simulink model "complete_model"  (R2020b)
settings: Solver=VariableStepAuto  StartTime=0.0  StopTime=10.0  RelTol=1e-3
undefined symbols (not defined in the file or in its folder): D_b_1, D_b_2, D_k_1, D_k_2, D_t_1, D_t_2, E_1, E_2, g, Gs_1, Gs_2, Ix_1, Ix_2, Iy_1, Iy_2, Iz_1, Iz_2, l_1, l_2, m_1, m_2, q_0, q_dot_0
libraries: dspmtrx3 x2, pid_lib x1, dspinverses x1
(part 2 of 2)

== matlab function complete_model/CONTROLLER/Subsystem2/MATLAB Function2 ==
  data: g input; B_matrix output; Ix_1 input; Ix_2 input; Iy_1 input; Iy_2 input; Iz_1 input; Iz_2 input; b_1 input; b_2 input; b_dot_1 input; b_dot_2 input; k_1 input; k_2 input; k_dot_1 input; k_dot_2 input; l_1 input; l_2 input; m_1 input; m_2 input; t_1 input; t_2 input; t_dot_1 input; t_dot_2 input; E_1 input; E_2 input; Gs_1 input; Gs_2 input; G_matrix output; C_matrix output
function [B_matrix,G_matrix,C_matrix] = compute_matrixs(g,Ix_1,Ix_2,Iy_1,Iy_2,Iz_1,Iz_2,b_1,b_2,b_dot_1,b_dot_2,k_1,k_2,k_dot_1,k_dot_2,l_1,l_2,m_1,m_2,t_1,t_2,t_dot_1,t_dot_2,E_1,E_2,Gs_1,Gs_2)

C_11 = C11(Ix_1,Iy_1,Iz_1,b_1,b_2,b_dot_1,b_dot_2,k_1,k_2,k_dot_1,k_dot_2,l_1,l_2,m_1,t_1,t_2,t_dot_1,t_dot_2);
C_12 = C12(Ix_1,Iy_1,Iz_1,b_1,b_2,b_dot_1,b_dot_2,k_1,k_2,k_dot_1,k_dot_2,l_1,l_2,m_1,t_1,t_2,t_dot_1,t_dot_2);
C_13 = C13(Ix_1,Iy_1,Iz_1,b_1,b_2,b_dot_1,b_dot_2,k_1,k_2,k_dot_1,k_dot_2,l_1,l_2,m_1,t_1,t_2,t_dot_1,t_dot_2);
C_14 = C14(Ix_1,Ix_2,Iy_1,Iy_2,Iz_1,Iz_2,b_1,b_2,b_dot_1,b_dot_2,k_1,k_2,k_dot_1,k_dot_2,l_1,l_2,m_1,m_2,t_1,t_2,t_dot_1,t_dot_2);
C_15 = C15(Ix_1,Ix_2,Iy_1,Iy_2,Iz_1,Iz_2,b_1,b_2,b_dot_1,b_dot_2,k_1,k_2,k_dot_1,k_dot_2,l_1,l_2,m_1,m_2,t_1,t_2,t_dot_1,t_dot_2);
C_16 = C16(Ix_1,Ix_2,Iy_1,Iy_2,Iz_1,Iz_2,b_1,b_2,b_dot_1,b_dot_2,k_1,k_2,k_dot_1,k_dot_2,l_1,l_2,m_1,m_2,t_1,t_2,t_dot_1,t_dot_2);

C_21 = C21(Ix_1,Iy_1,Iz_1,b_1,b_2,b_dot_1,b_dot_2,k_1,k_2,k_dot_1,k_dot_2,l_1,l_2,m_1,t_1,t_2,t_dot_1,t_dot_2);
C_22 = C22(Ix_1,Iy_1,Iz_1,b_1,b_2,b_dot_1,b_dot_2,k_1,k_2,k_dot_1,k_dot_2,l_1,l_2,m_1,t_1,t_2,t_dot_1,t_dot_2);
C_23 = C23(Ix_1,Iy_1,Iz_1,b_1,b_2,b_dot_1,b_dot_2,k_1,k_2,k_dot_1,k_dot_2,l_1,l_2,m_1,t_1,t_2,t_dot_1,t_dot_2);
C_24 = C24(Ix_1,Ix_2,Iy_1,Iy_2,Iz_1,Iz_2,b_1,b_2,b_dot_1,b_dot_2,k_1,k_2,k_dot_1,k_dot_2,l_1,l_2,m_1,m_2,t_1,t_2,t_dot_1,t_dot_2);
C_25 = C25(Ix_1,Ix_2,Iy_1,Iy_2,Iz_1,Iz_2,b_1,b_2,b_dot_1,b_dot_2,k_1,k_2,k_dot_1,k_dot_2,l_1,l_2,m_1,m_2,t_1,t_2,t_dot_1,t_dot_2);
C_26 = C26(Ix_1,Ix_2,Iy_1,Iy_2,Iz_1,Iz_2,b_1,b_2,b_dot_1,b_dot_2,k_1,k_2,k_dot_1,k_dot_2,l_1,l_2,m_1,m_2,t_1,t_2,t_dot_1,t_dot_2);

C_31 = C31(Ix_1,Iy_1,Iz_1,b_1,b_2,b_dot_1,b_dot_2,k_1,k_2,k_dot_1,k_dot_2,l_1,l_2,m_1,t_1,t_2,t_dot_1,t_dot_2);
C_32 = C32(Ix_1,Iy_1,Iz_1,b_1,b_2,b_dot_1,b_dot_2,k_1,k_2,k_dot_1,k_dot_2,l_1,l_2,m_1,t_1,t_2,t_dot_1,t_dot_2);
C_33 = C33(Ix_1,Iy_1,Iz_1,b_1,b_2,b_dot_1,b_dot_2,k_1,k_2,k_dot_1,k_dot_2,l_1,l_2,m_1,t_1,t_2,t_dot_1,t_dot_2);
C_34 = C34(Ix_1,Ix_2,Iy_1,Iy_2,Iz_1,Iz_2,b_1,b_2,b_dot_1,b_dot_2,k_1,k_2,k_dot_1,k_dot_2,l_1,l_2,m_1,m_2,t_1,t_2,t_dot_1,t_dot_2);
C_35 = C35(Ix_1,Ix_2,Iy_1,Iy_2,Iz_1,Iz_2,b_1,b_2,b_dot_1,b_dot_2,k_1,k_2,k_dot_1,k_dot_2,l_1,l_2,m_1,m_2,t_1,t_2,t_dot_1,t_dot_2);
C_36 = C36(Ix_1,Ix_2,Iy_1,Iy_2,Iz_1,Iz_2,b_1,b_2,b_dot_1,b_dot_2,k_1,k_2,k_dot_1,k_dot_2,l_1,l_2,m_1,m_2,t_1,t_2,t_dot_1,t_dot_2);

C_41 = C41(Ix_1,Ix_2,Iy_1,Iy_2,Iz_1,Iz_2,b_1,b_2,b_dot_1,b_dot_2,k_1,k_2,k_dot_1,k_dot_2,l_1,l_2,m_1,m_2,t_1,t_2,t_dot_1,t_dot_2);
C_42 = C42(Ix_1,Ix_2,Iy_1,Iy_2,Iz_1,Iz_2,b_1,b_2,b_dot_1,b_dot_2,k_1,k_2,k_dot_1,k_dot_2,l_1,l_2,m_1,m_2,t_1,t_2,t_dot_1,t_dot_2);
C_43 = C43(Ix_1,Ix_2,Iy_1,Iy_2,Iz_1,Iz_2,b_1,b_2,b_dot_1,b_dot_2,k_1,k_2,k_dot_1,k_dot_2,l_1,l_2,m_1,m_2,t_1,t_2,t_dot_1,t_dot_2);
C_44 = C44(Ix_2,Iy_2,Iz_2,b_1,b_2,b_dot_1,b_dot_2,k_1,k_2,k_dot_1,k_dot_2,l_1,l_2,m_2,t_1,t_2,t_dot_1,t_dot_2);
C_45 = C45(Ix_2,Iy_2,Iz_2,b_1,b_2,b_dot_1,b_dot_2,k_1,k_2,k_dot_1,k_dot_2,l_1,l_2,m_2,t_1,t_2,t_dot_1,t_dot_2);
C_46 = C46(Ix_2,Iy_2,Iz_2,b_1,b_2,b_dot_1,b_dot_2,k_1,k_2,k_dot_1,k_dot_2,l_1,l_2,m_2,t_1,t_2,t_dot_1,t_dot_2);

C_51 = C51(Ix_1,Ix_2,Iy_1,Iy_2,Iz_1,Iz_2,b_1,b_2,b_dot_1,b_dot_2,k_1,k_2,k_dot_1,k_dot_2,l_1,l_2,m_1,m_2,t_1,t_2,t_dot_1,t_dot_2);
C_52 = C52(Ix_1,Ix_2,Iy_1,Iy_2,Iz_1,Iz_2,b_1,b_2,b_dot_1,b_dot_2,k_1,k_2,k_dot_1,k_dot_2,l_1,l_2,m_1,m_2,t_1,t_2,t_dot_1,t_dot_2);
C_53 = C53(Ix_1,Ix_2,Iy_1,Iy_2,Iz_1,Iz_2,b_1,b_2,b_dot_1,b_dot_2,k_1,k_2,k_dot_1,k_dot_2,l_1,l_2,m_1,m_2,t_1,t_2,t_dot_1,t_dot_2);
C_54 = C54(Ix_2,Iy_2,Iz_2,b_1,b_2,b_dot_1,b_dot_2,k_1,k_2,k_dot_1,k_dot_2,l_1,l_2,m_2,t_1,t_2,t_dot_1,t_dot_2);
C_55 = C55(Ix_2,Iy_2,Iz_2,b_1,b_2,b_dot_1,b_dot_2,k_1,k_2,k_dot_1,k_dot_2,l_1,l_2,m_2,t_1,t_2,t_dot_1,t_dot_2);
C_56 = C56(Ix_2,Iy_2,Iz_2,b_1,b_2,b_dot_1,b_dot_2,k_1,k_2,k_dot_1,k_dot_2,l_1,l_2,m_2,t_1,t_2,t_dot_1,t_dot_2);

C_61 = C61(Ix_1,Ix_2,Iy_1,Iy_2,Iz_1,Iz_2,b_1,b_2,b_dot_1,b_dot_2,k_1,k_2,k_dot_1,k_dot_2,l_1,l_2,m_1,m_2,t_1,t_2,t_dot_1,t_dot_2);
C_62 = C62(Ix_1,Ix_2,Iy_1,Iy_2,Iz_1,Iz_2,b_1,b_2,b_dot_1,b_dot_2,k_1,k_2,k_dot_1,k_dot_2,l_1,l_2,m_1,m_2,t_1,t_2,t_dot_1,t_dot_2);
C_63 = C63(Ix_1,Ix_2,Iy_1,Iy_2,Iz_1,Iz_2,b_1,b_2,b_dot_1,b_dot_2,k_1,k_2,k_dot_1,k_dot_2,l_1,l_2,m_1,m_2,t_1,t_2,t_dot_1,t_dot_2);
C_64 = C64(Ix_2,Iy_2,Iz_2,b_1,b_2,b_dot_1,b_dot_2,k_1,k_2,k_dot_1,k_dot_2,l_1,l_2,m_2,t_1,t_2,t_dot_1,t_dot_2);
C_65 = C65(Ix_2,Iy_2,Iz_2,b_1,b_2,b_dot_1,b_dot_2,k_1,k_2,k_dot_1,k_dot_2,l_1,l_2,m_2,t_1,t_2,t_dot_1,t_dot_2);
C_66 = C66(Ix_2,Iy_2,Iz_2,b_1,b_2,b_dot_1,b_dot_2,k_1,k_2,k_dot_1,k_dot_2,l_1,l_2,m_2,t_1,t_2,t_dot_1,t_dot_2);

B_matrix = B(Ix_1,Ix_2,Iy_1,Iy_2,Iz_1,Iz_2,b_1,b_2,k_1,k_2,l_1,l_2,m_1,m_2,t_1,t_2);
G_matrix = G(E_1,E_2,Gs_1,Gs_2,Ix_1,Ix_2,Iy_1,Iy_2,Iz_1,Iz_2,b_1,b_2,g,k_1,k_2,l_1,l_2,m_1,m_2,t_1,t_2);
C_matrix = [    C_11 , C_12, C_13 , C_14 , C_15 , C_16 ;
                C_21 , C_22, C_23 , C_24 , C_25 , C_26 ;
                C_31 , C_32, C_33 , C_34 , C_35 , C_36 ;
                C_41 , C_42, C_43 , C_44 , C_45 , C_46 ;
                C_51 , C_52, C_53 , C_54 , C_55 , C_56 ;
                C_61 , C_62, C_63 , C_64 , C_65 , C_66 ;
                ];
            
end

== matlab function complete_model/ROBOT/Subsystem/MATLAB Function ==
  data: b_1 input; b_2 input; k_1 input; k_2 input; l_1 input; l_2 input; t_1 input; t_2 input; W_1 input; u output; W_2 input
function u = fcn( b_1,b_2,k_1,k_2,l_1,l_2,t_1,t_2,W_1, W_2)
    u_1 = J_1(b_1,b_2,k_1,k_2,l_1,l_2,t_1,t_2)' * W_1;
    u_2 = J_2(b_1,b_2,k_1,k_2,l_1,l_2,t_1,t_2)' * W_2;
    u = [u_1;u_2];

== matlab function complete_model/ROBOT/Subsystem1/MATLAB Function ==
  data: inv_B input; q_ddot output; C input; D input; G input; q_dot input; q input; u input
function q_ddot = fcn(inv_B,C,D,G,q_dot,q,u)
    q_ddot = - inv_B * ( C * q_dot + G + u + D * q_dot);

== matlab function complete_model/ROBOT/Subsystem/MATLAB Function2 ==
  data: g input; B_matrix output; Ix_1 input; Ix_2 input; Iy_1 input; Iy_2 input; Iz_1 input; Iz_2 input; b_1 input; b_2 input; b_dot_1 input; b_dot_2 input; k_1 input; k_2 input; k_dot_1 input; k_dot_2 input; l_1 input; l_2 input; m_1 input; m_2 input; t_1 input; t_2 input; t_dot_1 input; t_dot_2 input; E_1 input; E_2 input; Gs_1 input; Gs_2 input; G_matrix output; C_matrix output
function [B_matrix,G_matrix,C_matrix] = compute_matrixs(g,Ix_1,Ix_2,Iy_1,Iy_2,Iz_1,Iz_2,b_1,b_2,b_dot_1,b_dot_2,k_1,k_2,k_dot_1,k_dot_2,l_1,l_2,m_1,m_2,t_1,t_2,t_dot_1,t_dot_2,E_1,E_2,Gs_1,Gs_2)

C_11 = C11(Ix_1,Iy_1,Iz_1,b_1,b_2,b_dot_1,b_dot_2,k_1,k_2,k_dot_1,k_dot_2,l_1,l_2,m_1,t_1,t_2,t_dot_1,t_dot_2);
C_12 = C12(Ix_1,Iy_1,Iz_1,b_1,b_2,b_dot_1,b_dot_2,k_1,k_2,k_dot_1,k_dot_2,l_1,l_2,m_1,t_1,t_2,t_dot_1,t_dot_2);
C_13 = C13(Ix_1,Iy_1,Iz_1,b_1,b_2,b_dot_1,b_dot_2,k_1,k_2,k_dot_1,k_dot_2,l_1,l_2,m_1,t_1,t_2,t_dot_1,t_dot_2);
C_14 = C14(Ix_1,Ix_2,Iy_1,Iy_2,Iz_1,Iz_2,b_1,b_2,b_dot_1,b_dot_2,k_1,k_2,k_dot_1,k_dot_2,l_1,l_2,m_1,m_2,t_1,t_2,t_dot_1,t_dot_2);
C_15 = C15(Ix_1,Ix_2,Iy_1,Iy_2,Iz_1,Iz_2,b_1,b_2,b_dot_1,b_dot_2,k_1,k_2,k_dot_1,k_dot_2,l_1,l_2,m_1,m_2,t_1,t_2,t_dot_1,t_dot_2);
C_16 = C16(Ix_1,Ix_2,Iy_1,Iy_2,Iz_1,Iz_2,b_1,b_2,b_dot_1,b_dot_2,k_1,k_2,k_dot_1,k_dot_2,l_1,l_2,m_1,m_2,t_1,t_2,t_dot_1,t_dot_2);

C_21 = C21(Ix_1,Iy_1,Iz_1,b_1,b_2,b_dot_1,b_dot_2,k_1,k_2,k_dot_1,k_dot_2,l_1,l_2,m_1,t_1,t_2,t_dot_1,t_dot_2);
C_22 = C22(Ix_1,Iy_1,Iz_1,b_1,b_2,b_dot_1,b_dot_2,k_1,k_2,k_dot_1,k_dot_2,l_1,l_2,m_1,t_1,t_2,t_dot_1,t_dot_2);
C_23 = C23(Ix_1,Iy_1,Iz_1,b_1,b_2,b_dot_1,b_dot_2,k_1,k_2,k_dot_1,k_dot_2,l_1,l_2,m_1,t_1,t_2,t_dot_1,t_dot_2);
C_24 = C24(Ix_1,Ix_2,Iy_1,Iy_2,Iz_1,Iz_2,b_1,b_2,b_dot_1,b_dot_2,k_1,k_2,k_dot_1,k_dot_2,l_1,l_2,m_1,m_2,t_1,t_2,t_dot_1,t_dot_2);
C_25 = C25(Ix_1,Ix_2,Iy_1,Iy_2,Iz_1,Iz_2,b_1,b_2,b_dot_1,b_dot_2,k_1,k_2,k_dot_1,k_dot_2,l_1,l_2,m_1,m_2,t_1,t_2,t_dot_1,t_dot_2);
C_26 = C26(Ix_1,Ix_2,Iy_1,Iy_2,Iz_1,Iz_2,b_1,b_2,b_dot_1,b_dot_2,k_1,k_2,k_dot_1,k_dot_2,l_1,l_2,m_1,m_2,t_1,t_2,t_dot_1,t_dot_2);

C_31 = C31(Ix_1,Iy_1,Iz_1,b_1,b_2,b_dot_1,b_dot_2,k_1,k_2,k_dot_1,k_dot_2,l_1,l_2,m_1,t_1,t_2,t_dot_1,t_dot_2);
C_32 = C32(Ix_1,Iy_1,Iz_1,b_1,b_2,b_dot_1,b_dot_2,k_1,k_2,k_dot_1,k_dot_2,l_1,l_2,m_1,t_1,t_2,t_dot_1,t_dot_2);
C_33 = C33(Ix_1,Iy_1,Iz_1,b_1,b_2,b_dot_1,b_dot_2,k_1,k_2,k_dot_1,k_dot_2,l_1,l_2,m_1,t_1,t_2,t_dot_1,t_dot_2);
C_34 = C34(Ix_1,Ix_2,Iy_1,Iy_2,Iz_1,Iz_2,b_1,b_2,b_dot_1,b_dot_2,k_1,k_2,k_dot_1,k_dot_2,l_1,l_2,m_1,m_2,t_1,t_2,t_dot_1,t_dot_2);
C_35 = C35(Ix_1,Ix_2,Iy_1,Iy_2,Iz_1,Iz_2,b_1,b_2,b_dot_1,b_dot_2,k_1,k_2,k_dot_1,k_dot_2,l_1,l_2,m_1,m_2,t_1,t_2,t_dot_1,t_dot_2);
C_36 = C36(Ix_1,Ix_2,Iy_1,Iy_2,Iz_1,Iz_2,b_1,b_2,b_dot_1,b_dot_2,k_1,k_2,k_dot_1,k_dot_2,l_1,l_2,m_1,m_2,t_1,t_2,t_dot_1,t_dot_2);

C_41 = C41(Ix_1,Ix_2,Iy_1,Iy_2,Iz_1,Iz_2,b_1,b_2,b_dot_1,b_dot_2,k_1,k_2,k_dot_1,k_dot_2,l_1,l_2,m_1,m_2,t_1,t_2,t_dot_1,t_dot_2);
C_42 = C42(Ix_1,Ix_2,Iy_1,Iy_2,Iz_1,Iz_2,b_1,b_2,b_dot_1,b_dot_2,k_1,k_2,k_dot_1,k_dot_2,l_1,l_2,m_1,m_2,t_1,t_2,t_dot_1,t_dot_2);
C_43 = C43(Ix_1,Ix_2,Iy_1,Iy_2,Iz_1,Iz_2,b_1,b_2,b_dot_1,b_dot_2,k_1,k_2,k_dot_1,k_dot_2,l_1,l_2,m_1,m_2,t_1,t_2,t_dot_1,t_dot_2);
C_44 = C44(Ix_2,Iy_2,Iz_2,b_1,b_2,b_dot_1,b_dot_2,k_1,k_2,k_dot_1,k_dot_2,l_1,l_2,m_2,t_1,t_2,t_dot_1,t_dot_2);
C_45 = C45(Ix_2,Iy_2,Iz_2,b_1,b_2,b_dot_1,b_dot_2,k_1,k_2,k_dot_1,k_dot_2,l_1,l_2,m_2,t_1,t_2,t_dot_1,t_dot_2);
C_46 = C46(Ix_2,Iy_2,Iz_2,b_1,b_2,b_dot_1,b_dot_2,k_1,k_2,k_dot_1,k_dot_2,l_1,l_2,m_2,t_1,t_2,t_dot_1,t_dot_2);

C_51 = C51(Ix_1,Ix_2,Iy_1,Iy_2,Iz_1,Iz_2,b_1,b_2,b_dot_1,b_dot_2,k_1,k_2,k_dot_1,k_dot_2,l_1,l_2,m_1,m_2,t_1,t_2,t_dot_1,t_dot_2);
C_52 = C52(Ix_1,Ix_2,Iy_1,Iy_2,Iz_1,Iz_2,b_1,b_2,b_dot_1,b_dot_2,k_1,k_2,k_dot_1,k_dot_2,l_1,l_2,m_1,m_2,t_1,t_2,t_dot_1,t_dot_2);
C_53 = C53(Ix_1,Ix_2,Iy_1,Iy_2,Iz_1,Iz_2,b_1,b_2,b_dot_1,b_dot_2,k_1,k_2,k_dot_1,k_dot_2,l_1,l_2,m_1,m_2,t_1,t_2,t_dot_1,t_dot_2);
C_54 = C54(Ix_2,Iy_2,Iz_2,b_1,b_2,b_dot_1,b_dot_2,k_1,k_2,k_dot_1,k_dot_2,l_1,l_2,m_2,t_1,t_2,t_dot_1,t_dot_2);
C_55 = C55(Ix_2,Iy_2,Iz_2,b_1,b_2,b_dot_1,b_dot_2,k_1,k_2,k_dot_1,k_dot_2,l_1,l_2,m_2,t_1,t_2,t_dot_1,t_dot_2);
C_56 = C56(Ix_2,Iy_2,Iz_2,b_1,b_2,b_dot_1,b_dot_2,k_1,k_2,k_dot_1,k_dot_2,l_1,l_2,m_2,t_1,t_2,t_dot_1,t_dot_2);

C_61 = C61(Ix_1,Ix_2,Iy_1,Iy_2,Iz_1,Iz_2,b_1,b_2,b_dot_1,b_dot_2,k_1,k_2,k_dot_1,k_dot_2,l_1,l_2,m_1,m_2,t_1,t_2,t_dot_1,t_dot_2);
C_62 = C62(Ix_1,Ix_2,Iy_1,Iy_2,Iz_1,Iz_2,b_1,b_2,b_dot_1,b_dot_2,k_1,k_2,k_dot_1,k_dot_2,l_1,l_2,m_1,m_2,t_1,t_2,t_dot_1,t_dot_2);
C_63 = C63(Ix_1,Ix_2,Iy_1,Iy_2,Iz_1,Iz_2,b_1,b_2,b_dot_1,b_dot_2,k_1,k_2,k_dot_1,k_dot_2,l_1,l_2,m_1,m_2,t_1,t_2,t_dot_1,t_dot_2);
C_64 = C64(Ix_2,Iy_2,Iz_2,b_1,b_2,b_dot_1,b_dot_2,k_1,k_2,k_dot_1,k_dot_2,l_1,l_2,m_2,t_1,t_2,t_dot_1,t_dot_2);
C_65 = C65(Ix_2,Iy_2,Iz_2,b_1,b_2,b_dot_1,b_dot_2,k_1,k_2,k_dot_1,k_dot_2,l_1,l_2,m_2,t_1,t_2,t_dot_1,t_dot_2);
C_66 = C66(Ix_2,Iy_2,Iz_2,b_1,b_2,b_dot_1,b_dot_2,k_1,k_2,k_dot_1,k_dot_2,l_1,l_2,m_2,t_1,t_2,t_dot_1,t_dot_2);

B_matrix = B(Ix_1,Ix_2,Iy_1,Iy_2,Iz_1,Iz_2,b_1,b_2,k_1,k_2,l_1,l_2,m_1,m_2,t_1,t_2);
G_matrix = G(E_1,E_2,Gs_1,Gs_2,Ix_1,Ix_2,Iy_1,Iy_2,Iz_1,Iz_2,b_1,b_2,g,k_1,k_2,l_1,l_2,m_1,m_2,t_1,t_2);
C_matrix = [    C_11 , C_12, C_13 , C_14 , C_15 , C_16 ;
                C_21 , C_22, C_23 , C_24 , C_25 , C_26 ;
                C_31 , C_32, C_33 , C_34 , C_35 , C_36 ;
                C_41 , C_42, C_43 , C_44 , C_45 , C_46 ;
                C_51 , C_52, C_53 , C_54 , C_55 , C_56 ;
                C_61 , C_62, C_63 , C_64 , C_65 , C_66 ;
                ];
            
end

== matlab function complete_model/CONTROL_TO_FORCE /Subsystem/MATLAB Function ==
  data: b_1 input; b_2 input; k_1 input; k_2 input; l_1 input; l_2 input; t_1 input; t_2 input; u_ctrl_1 input; W_ctrl_1 output; u_ctrl_2 input; W_ctrl_2 output
function [W_ctrl_1 , W_ctrl_2] = fcn( b_1,b_2,k_1,k_2,l_1,l_2,t_1,t_2,u_ctrl_1, u_ctrl_2)
%     J_p_1= pinv(J_1(b_1,b_2,k_1,k_2,l_1,l_2,t_1,t_2)' );
%     J_p_2 = pinv(J_2(b_1,b_2,k_1,k_2,l_1,l_2,t_1,t_2)' );
%     W_ctrl_1_p = J_p_1(4:6,1:3) * u_ctrl_1 ;
%     W_ctrl_2_p = J_p_2(4:6,1:3) * u_ctrl_2 ;
%     W_ctrl_1 = [0;0;0;W_ctrl_1_p]
%     W_ctrl_2 = [0;0;0;W_ctrl_2_p]
    J_p_1 = pinv(J_1(b_1,b_2,k_1,k_2,l_1,l_2,t_1,t_2) )' ;
    J_p_2 = pinv(J_2(b_1,b_2,k_1,k_2,l_1,l_2,t_1,t_2) )' ;
    W_ctrl_1 = J_p_1 * u_ctrl_1 ;
    W_ctrl_2 = J_p_2 * u_ctrl_2 ;
